simulink model "pair_harmonics"  (R2023b)
settings: Solver=FixedStepAuto  StartTime=0.0  StopTime=0.2  RelTol=1e-3
libraries: spsVoltageMeasurementLib x6, spsACVoltageSourceLib x4, spsCurrentMeasurementLib x3, spsGroundLib x3, dspstat3 x3, spsSeriesRLCBranchLib x3, spsVariableInductorLib x3, sps_lib x1
settings Model: Creator=enesa  LastModifiedBy=enesa

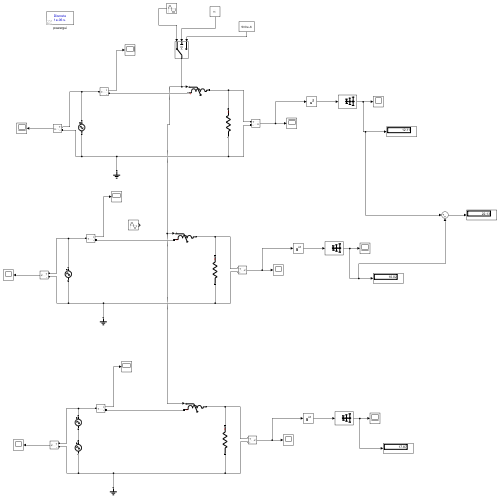
[thumbnail: Simulink's stored preview of the top-level diagram]
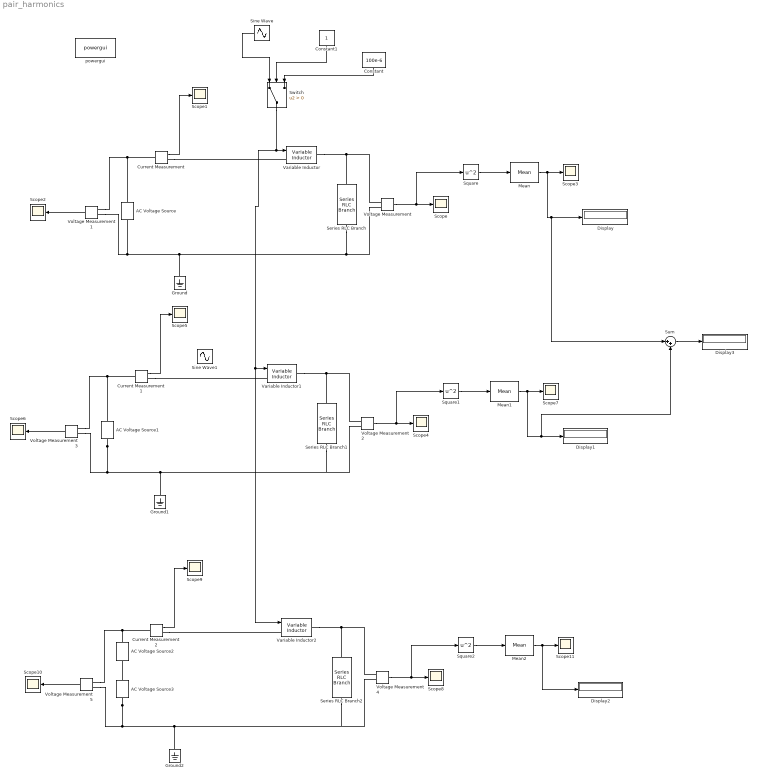
== system pair_harmonics ==
  AC Voltage Source : spsACVoltageSourceLib/AC Voltage Source  Amplitude=100  Phase=0  Frequency=10e3  SampleTime=0  Measurements=None  BusType=swing  Pref=10e3  Qref=0  Qmin=-inf  Qmax=+inf
  AC Voltage Source1 : spsACVoltageSourceLib/AC Voltage Source  Amplitude=100  Phase=0  Frequency=11e3  SampleTime=0  Measurements=None  BusType=swing  Pref=10e3  Qref=0  Qmin=-inf  Qmax=+inf
  AC Voltage Source2 : spsACVoltageSourceLib/AC Voltage Source  Amplitude=100  Phase=0  Frequency=11e3  SampleTime=0  Measurements=None  BusType=swing  Pref=10e3  Qref=0  Qmin=-inf  Qmax=+inf
  AC Voltage Source3 : spsACVoltageSourceLib/AC Voltage Source  Amplitude=100  Phase=0  Frequency=10e3  SampleTime=0  Measurements=None  BusType=swing  Pref=10e3  Qref=0  Qmin=-inf  Qmax=+inf
  Constant : Constant  Value=100e-6
  Constant1 : Constant
  Current Measurement : spsCurrentMeasurementLib/Current Measurement  PhasorSimulation=off  OutputType=Complex  PSBequivalent=0
  Current Measurement1 : spsCurrentMeasurementLib/Current Measurement  PhasorSimulation=off  OutputType=Complex  PSBequivalent=0
  Current Measurement2 : spsCurrentMeasurementLib/Current Measurement  PhasorSimulation=off  OutputType=Complex  PSBequivalent=0
  Display{,1..3} (4 alike) : Display
  Ground : spsGroundLib/Ground  LConnTagsString=a
  Ground1 : spsGroundLib/Ground  LConnTagsString=a
  Ground2 : spsGroundLib/Ground  LConnTagsString=a
  Mean : dspstat3/Mean  run=on  InputProcessing=Columns as channels (frame based)  reset_popup=None  directionMode=Each column  dimension=1  roiEnable=off  roiType=Rectangles  roiPortion=Entire ROI  roiOutput=Individual statistics for each ROI  roiFlag=off  roundingMode=Floor  overflowMode=off  outputDataTypeStr=Inherit: Same as accumulator  outputMin=[]  outputMax=[]  outputLastDataTypeStr=Inherit: Same as accumulator
  Mean1 : dspstat3/Mean  run=on  InputProcessing=Columns as channels (frame based)  reset_popup=None  directionMode=Each column  dimension=1  roiEnable=off  roiType=Rectangles  roiPortion=Entire ROI  roiOutput=Individual statistics for each ROI  roiFlag=off  roundingMode=Floor  overflowMode=off  outputDataTypeStr=Inherit: Same as accumulator  outputMin=[]  outputMax=[]  outputLastDataTypeStr=Inherit: Same as accumulator
  Mean2 : dspstat3/Mean  run=on  InputProcessing=Columns as channels (frame based)  reset_popup=None  directionMode=Each column  dimension=1  roiEnable=off  roiType=Rectangles  roiPortion=Entire ROI  roiOutput=Individual statistics for each ROI  roiFlag=off  roundingMode=Floor  overflowMode=off  outputDataTypeStr=Inherit: Same as accumulator  outputMin=[]  outputMax=[]  outputLastDataTypeStr=Inherit: Same as accumulator
  Scope{,1..11} (12 alike) : Scope
  Series RLC Branch : spsSeriesRLCBranchLib/Series RLC Branch  LConnTagsString=__new0  RConnTagsString=__new0  BranchType=R  Resistance=0.2  Inductance=1e-3  SetiL0=off  InitialCurrent=0  Capacitance=1e-6  Setx0=off  InitialVoltage=0  Measurements=None
  Series RLC Branch1 : spsSeriesRLCBranchLib/Series RLC Branch  LConnTagsString=__new0  RConnTagsString=__new0  BranchType=R  Resistance=0.2  Inductance=1e-3  SetiL0=off  InitialCurrent=0  Capacitance=1e-6  Setx0=off  InitialVoltage=0  Measurements=None
  Series RLC Branch2 : spsSeriesRLCBranchLib/Series RLC Branch  LConnTagsString=__new0  RConnTagsString=__new0  BranchType=R  Resistance=0.2  Inductance=1e-3  SetiL0=off  InitialCurrent=0  Capacitance=1e-6  Setx0=off  InitialVoltage=0  Measurements=None
  Sine Wave : Sin  Amplitude=40e-6  Bias=80e-6  Frequency=2*pi*500  SampleTime=0
  Sine Wave1 : Sin  Amplitude=20e-6  Bias=80e-6  Frequency=2*pi*500  SampleTime=0
  Square : Math  Operator=square
  Square1 : Math  Operator=square
  Square2 : Math  Operator=square
  Sum : Sum  Inputs=|++
  Switch : Switch  Criteria=u2 > Threshold  SaturateOnIntegerOverflow=off  InputSameDT=off
  Variable Inductor : spsVariableInductorLib/Variable Inductor  methode=Backward Euler  Labsmin=1e-6  Initialize=off  iL0=0  L0=1e-3  Vl0=0
      settings: LibrarySourceBlock=sps_lib/Passives/Variable Inductor
  Variable Inductor1 : spsVariableInductorLib/Variable Inductor  methode=Backward Euler  Labsmin=1e-6  Initialize=off  iL0=0  L0=1e-3  Vl0=0
      settings: LibrarySourceBlock=sps_lib/Passives/Variable Inductor
  Variable Inductor2 : spsVariableInductorLib/Variable Inductor  methode=Backward Euler  Labsmin=1e-6  Initialize=off  iL0=0  L0=1e-3  Vl0=0
      settings: LibrarySourceBlock=sps_lib/Passives/Variable Inductor
  Voltage Measurement{,1..5} (6 alike) : spsVoltageMeasurementLib/Voltage Measurement  PhasorSimulation=off  OutputType=Complex  PSBequivalent=0
  powergui : sps_lib/powergui  Priority=1  SimulationMode=Discrete  SampleTime=1e-6  frequency=60  Iterations=50  frequencyindice=0  Pbase=100e6  ErrMax=1e-4  UnitsV=kV  UnitsW=MW  buscounter=0  FunctionMessages=off  echomessages=off  EnableUseOfTLC=off  CurrentSourceSwitches=off  DisableSnubberDevices=off  DisableRonSwitches=off  DisableVfSwitches=off  DisplayEquations=off  AutomaticDiscreteSolvers=off  SolverType=Tustin/Backward Euler (TBE)  Interpol=off  ExternalGateDelay=off  methode=off  Ts=100  x0status=blocks  SPID=on  SwTol=0  HookPort=off  NonlinearTolerance=1e-4  nMaxIteration=100  ContinueOnMaxIteration=off  RestoreLinks=warning  ResistiveCurrentMeasurement=off  Frange=[0:2:500]  Ylog=off  Xlog=on  ShowGrid=off  save=off  variable=ZData  structure=0  ZoomFFT=off  StartTime=0.0  cycles=1  DisplayStyle=1  fundamental=60  FreqAxis=off  MaxFrequency=1000  frequencyindicesteady=1  RmsSteady=1  display=off
  wires:
  Current Measurement/1 -> Scope1/1
  Voltage Measurement1/1 -> Scope2/1
  Sine Wave/1 -> Switch/1
  Voltage Measurement/1 -> Square/1, Scope/1
  Square/1 -> Mean/1
  Mean/1 -> Sum/1, Display/1, Scope3/1
  Square1/1 -> Mean1/1
  Mean1/1 -> Sum/2, Display1/1, Scope7/1
  Current Measurement1/1 -> Scope5/1
  Voltage Measurement2/1 -> Square1/1, Scope4/1
  Voltage Measurement3/1 -> Scope6/1
  Mean2/1 -> Display2/1, Scope11/1
  Current Measurement2/1 -> Scope9/1
  Square2/1 -> Mean2/1
  Voltage Measurement4/1 -> Square2/1, Scope8/1
  Voltage Measurement5/1 -> Scope10/1
  Sum/1 -> Display3/1
  Constant/1 -> Switch/3
  Switch/1 -> Variable Inductor2/1, Variable Inductor1/1, Variable Inductor/1
  Constant1/1 -> Switch/2
  connections:
  Current Measurement/LConn1 -- AC Voltage Source/RConn1 -- Voltage Measurement1/LConn1
  Variable Inductor/RConn1 -- Series RLC Branch/LConn1 -- Voltage Measurement/LConn1
  Series RLC Branch/RConn1 -- Voltage Measurement/LConn2 -- Ground/LConn1 -- Voltage Measurement1/LConn2 -- AC Voltage Source/LConn1
  Current Measurement/RConn1 -- Variable Inductor/LConn1
  AC Voltage Source1/LConn1 -- Ground1/LConn1 -- Series RLC Branch1/RConn1 -- Voltage Measurement2/LConn2 -- Voltage Measurement3/LConn2
  Voltage Measurement3/LConn1 -- AC Voltage Source1/RConn1 -- Current Measurement1/LConn1
  Voltage Measurement2/LConn1 -- Series RLC Branch1/LConn1 -- Variable Inductor1/RConn1
  Current Measurement1/RConn1 -- Variable Inductor1/LConn1
  AC Voltage Source3/LConn1 -- Ground2/LConn1 -- Series RLC Branch2/RConn1 -- Voltage Measurement4/LConn2 -- Voltage Measurement5/LConn2
  Voltage Measurement4/LConn1 -- Series RLC Branch2/LConn1 -- Variable Inductor2/RConn1
  Voltage Measurement5/LConn1 -- AC Voltage Source2/RConn1 -- Current Measurement2/LConn1
  Current Measurement2/RConn1 -- Variable Inductor2/LConn1
  AC Voltage Source3/RConn1 -- AC Voltage Source2/LConn1
